simulink model "OpenSeesPy_Raspberry"  (R2021a)
settings: Solver=ode8  StartTime=0.0  StopTime=31.2  FixedStep=dtfast  RelTol=1e-3
PreLoadFcn:
  | initializeSimulation;
InitFcn:
  | clear('all');
  | initializeSimulation;
undefined symbols (not defined in the file): adaptive, Area, asiv, Be, Cl, denfilter, DiscIntNeverNeededParam, dtsim, fir_coef, forgfact, Gsnsr_DT, Gsnsr_FT, Kc, ke, kgap, khard, Kp, Kq, kv, learningrate, n1siv, n2siv, Ngap, nsiv, numfilter, P_corr_i, Seed_snr, ssAe, ssBe, ssCe, ssDe, stiffdeg, strdegHmos, tauv, V1, Vt, w_80, x02, xgap, xy
libraries: simulink x4, raspberrypiNetworklib x2
settings Model: Creator=diego.mera  LastModifiedBy=diego.mera
settings SolverCC: PositivePriorityOrder=on
settings OptimizationCC: EnhancedBackFolding=on  PassReuseOutputArgsAs=Individual arguments  ZeroExternalMemoryAtStartup=off  ZeroInternalMemoryAtStartup=off  MaxStackSize=64  OptimizeBlockOrder=speed  DifferentSizesBufferReuse=on  OptimizationCustomize=off  EfficientTunableParamExpr=on
settings DebuggingCC: ParameterTunabilityLossMsg=error
settings HardwareCC: ProdBitPerPointer=32  ProdBitPerSizeT=32  ProdBitPerPtrDiffT=32  ProdLargestAtomicInteger=Long  ProdLargestAtomicFloat=Double  ProdWordSize=32  ProdLongLongMode=on  ProdHWDeviceType=ARM Compatible->ARM Cortex
settings RTWCC: SystemTargetFile=ert.tlc  HardwareBoard=Raspberry Pi  TLCOptions="-aInlineSetEventsForThisBaseRateFcn=TLC_FALSE -aSuppressMultiTaskScheduler=TLC_FALSE  -aRateBasedStepFcn=0"  TemplateMakefile=ert_default_tmf  Toolchain=GNU GCC Embedded Linux  BuildConfiguration=Faster Runs
settings CodeAppCC: ForceParamTrailComments=on  IgnoreCustomStorageClasses=off  OperatorAnnotations=on  SimulinkDataObjDesc=on  SFDataObjDesc=on  InsertBlockDesc=on
settings ERTTargetCC: SupportContinuousTime=on  SupportVariableSizeSignals=on  ExtModeTransport=2  ExtModeStaticAlloc=on  ExtModeMexFile=ext_xcp  ExtModeIntrfLevel=Level2 - Open

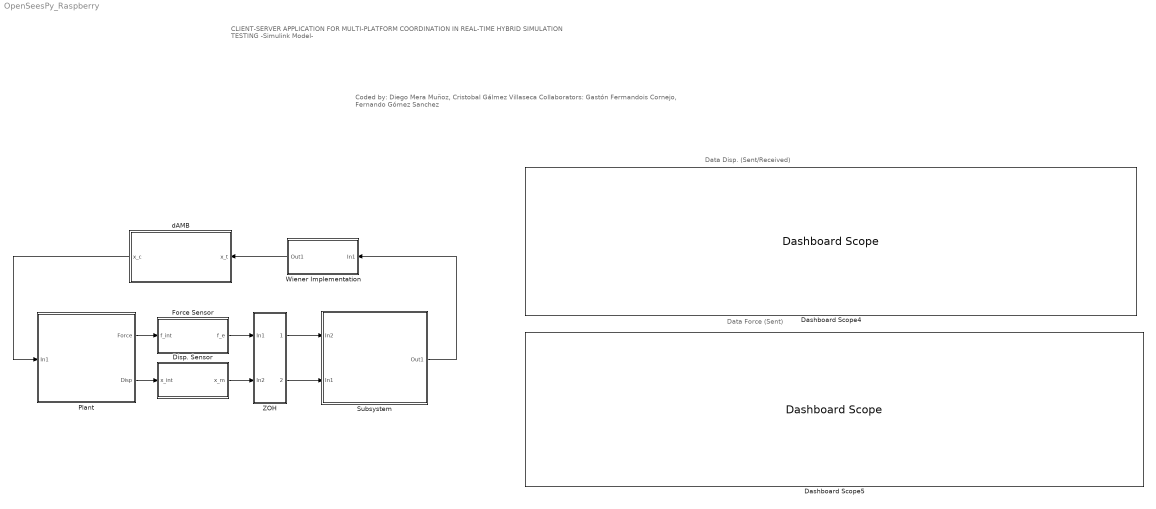
== system OpenSeesPy_Raspberry ==
  note: Data Disp. (Sent/Received)
  note: Data Force (Sent)
  note: Coded by: Diego Mera Muñoz, Cristobal Gálmez Villaseca
      | Collaborators: Gastón Fermandois Cornejo, Fernando Gómez Sanchez
  note: CLIENT-SERVER APPLICATION FOR MULTI-PLATFORM COORDINATION IN REAL-TIME HYBRID SIMULATION TESTING
      | -Simulink Model-
  Dashboard Scope4 : DashboardScope  Ymin=-5  Ymax=5
  Dashboard Scope5 : DashboardScope  Ymin=-1.5e-5  Ymax=1e-5
  Disp. Sensor : Subsystem
      mask Display: disp('DISP. SENSOR')
  Force Sensor : Subsystem
      mask Display: disp('FORCE SENSOR')
  Plant : Subsystem
      mask Display: disp('PLANT\n(Actuator-ES)')
  Subsystem : Subsystem
      mask Display: disp('NUMERICAL\nSUBSTRUCTURE')
  Wiener Implementation : Subsystem
      mask Display: disp('MBMRT FILTER')
  ZOH : Subsystem
      mask Display: disp('ZOH')
  dAMB : Subsystem
      mask Display: disp('DISCRETE ADAPTIVE\nMODEL-BASED\nCOMPENSATION')
  wires:
  Subsystem/1(Out1) -> Wiener Implementation/1(In1)
  Wiener Implementation/1(Out1) -> dAMB/1(x_t)
  Plant/1(Force) -> Force Sensor/1(f_int)
  Plant/2(Disp) -> Disp. Sensor/1(x_int)
  dAMB/1(x_c) -> Plant/1(In1)
  ZOH/1(Out1) -> Subsystem/1(In2)
  ZOH/2(Out2) -> Subsystem/2(In1)
  Force Sensor/1("f_e ") -> ZOH/1(In1)
  Disp. Sensor/1(x_m) -> ZOH/2(In2)

== system OpenSeesPy_Raspberry/Disp. Sensor ==
  x_int : Inport
  Sensor Noise : simulink/Sources/Band-Limited White Noise  Cov=rms_noise_DT  Ts=dtsim  seed=double(Seed_snr.Seed)
  Sensor Gain LVDT : Gain  Gain=Gsnsr_DT  SaturateOnIntegerOverflow=on  OutDataTypeStr=Inherit: Same as input  ParamDataTypeStr=Inherit: Same as input
  Sum : Sum  Inputs=|++  InputSameDT=on  SaturateOnIntegerOverflow=on  OutDataTypeStr=Inherit: Same as first input
  x_m : Outport
  tag scope: x_m=global
  wires:
  Sensor Noise/1 -> Sum/2
  Sum/1 -> x_m/1, [x_m]  "x_m"
  x_int/1 -> Sensor Gain LVDT/1
  Sensor Gain LVDT/1 -> Sum/1

== system OpenSeesPy_Raspberry/Force Sensor ==
  f_int : Inport
  Sensor Noise1 : simulink/Sources/Band-Limited White Noise  Cov=rms_noise_FT  Ts=dtsim  seed=double(Seed_snr.Seed)
  Sensor Gain LOAD CELL : Gain  Gain=Gsnsr_FT  SaturateOnIntegerOverflow=on  OutDataTypeStr=Inherit: Same as input  ParamDataTypeStr=Inherit: Same as input
  Sum1 : Sum  Inputs=|++  InputSameDT=on  SaturateOnIntegerOverflow=on  OutDataTypeStr=Inherit: Same as first input
  "f_e " : Outport
  wires:
  f_int/1 -> Sensor Gain LOAD CELL/1
  Sensor Noise1/1 -> Sum1/2
  Sum1/1 -> "f_e "/1
  Sensor Gain LOAD CELL/1 -> Sum1/1

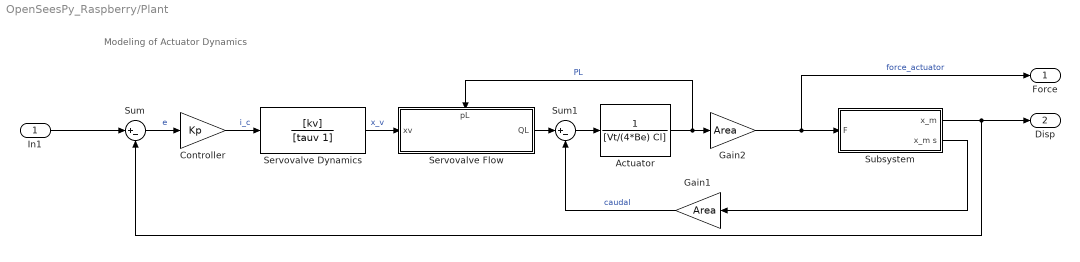
== system OpenSeesPy_Raspberry/Plant ==
  note: Modeling of Actuator Dynamics
  In1 : Inport
  Actuator : TransferFcn  Denominator=[Vt/(4*Be) Cl]
      mask Display: image(imread('actuator.PNG'));
  Controller : Gain  Gain=Kp
  Gain1 : Gain  Gain=Area
  Gain2 : Gain  Gain=Area
  Servovalve Dynamics : TransferFcn  Numerator=[kv]  Denominator=[tauv 1]
      mask Display: image(imread('servo2.PNG'));
  Servovalve Flow : Subsystem
      settings: PortSchema="{\"entries\":[{\"content\":{\"sides\":[{\"content\":{\"connectorIds\":[\"In1\"]},\"type\":\"ConnectorPlacement.EquallySpacedRectSide\",\"uuid\":\"f3a8b7d5-d784-462c-bc82-60644eee5a75\"},{\"content\":{\"connectorIds\":[\"Out1\"],\"side\":\"RIGHT\"},\"type\":\"ConnectorPlacement.EquallySpacedRectSide\",\"uuid\":\"5e6f1f83-a632-4bc9-a761-43cae998e77f\"},{\"content\":{\"connectorIds\":[\"In2\"],\"side\":\"TOP\"},\"type\":\"ConnectorPlacement.EquallySpacedRectSide\",\"uuid\":\"989b0903-e260-4847-946f-0ac5d5e511f7\"}]},\"type\":\"ConnectorPlacement.EquallySpacedConnector\",\"uuid\":\"5619e211-faa3-4076-b1a0-b20862ba0eaa\"}],\"packageUris\":[\"http://schema.mathworks.com/mf0/Connector/19700101\"],\"version\":\"1.0\"}"
      mask Display: image(imread('servo.PNG'));
  Subsystem : Subsystem
      mask Display: disp('EXPERIMENTAL\nSUBSTRUCTURE')
  Sum : Sum  Inputs=|+-
  Sum1 : Sum  Inputs=|+-
  Force : Outport
  Disp : Outport  Port=2
  wires:
  Sum/1 -> Controller/1  "e"
  Servovalve Dynamics/1 -> Servovalve Flow/1(xv)  "x_v"
  Gain1/1 -> Sum1/2  "caudal"
  Actuator/1 -> Servovalve Flow/2(pL), Gain2/1  "PL"
  Sum1/1 -> Actuator/1
  Controller/1 -> Servovalve Dynamics/1  "i_c"
  Servovalve Flow/1(QL) -> Sum1/1
  Gain2/1 -> Subsystem/1(F), Force/1  "force_actuator"
  Subsystem/2(x_m s) -> Gain1/1
  Subsystem/1(x_m) -> Disp/1, Sum/2
  In1/1 -> Sum/1

== system OpenSeesPy_Raspberry/Subsystem ==
  In2 : Inport
  In1 : Inport  Port=2
  Display10 : Display
  TCP/IP Receive2 : raspberrypiNetworklib/TCP//IP Receive  Priority=2  Mode_=Client  LocalServerPort_=8090  RemoteAddr_=192.168.0.18  RemoteServerPort_=8090  DataType_=double  DataSize_=1  SampleTime_=dtsim  SimulateUsing=Code generation  ClientPortBindingSelection_=off  ClientPortToBind_=35000  BlockingMode_=on  BlockTimeout_=0.01  BlockPlatform=RASPBERRYPI
      settings: SourceProductBaseCode=RASPPI
  TCP/IP Send1 : raspberrypiNetworklib/TCP//IP Send  Priority=1  Mode_=Client  LocalServerPort_=8090  RemoteAddr_=192.168.0.18  RemoteServerPort_=8090  SimulateUsing=Code generation  ClientPortBindingSelection_=off  ClientPortToBind_=35000  BlockingMode_=on  BlockTimeout_=0.02  BlockPlatform=RASPBERRYPI
      settings: SourceProductBaseCode=RASPPI
  Terminator : Terminator
  Out1 : Outport
  wires:
  In1/1 -> Terminator/1
  In2/1 -> TCP/IP Send1/1  "Disp_Num"
  TCP/IP Receive2/1 -> Out1/1
  TCP/IP Receive2/2 -> Display10/1

== system OpenSeesPy_Raspberry/Wiener Implementation ==
  In1 : Inport
  Prediction_Fixed_Adaptive : Subsystem
      mask Display: disp('PREDICTION\n(Adaptive/Fixed w)')
  Test3 : Subsystem
      mask Display: disp('MONOMIAL\nINTERPOLATION')
  To Workspace : ToWorkspace  VariableName=adaptive_parameters  SaveFormat=Timeseries  SampleTime=-1
  Out1 : Outport
  wires:
  Prediction_Fixed_Adaptive/2(Out2) -> To Workspace/1
  Test3/1(Out1) -> Out1/1
  In1/1 -> Prediction_Fixed_Adaptive/1(In1)
  Prediction_Fixed_Adaptive/1(Out1) -> Test3/1(In1)

== system OpenSeesPy_Raspberry/ZOH ==
  In1 : Inport
  In2 : Inport  Port=2
  Rate Transition : RateTransition  OutPortSampleTime=dtsim
  Rate Transition1 : RateTransition  OutPortSampleTime=dtsim
  Out1 : Outport
  Out2 : Outport  Port=2
  wires:
  In1/1 -> Rate Transition/1
  In2/1 -> Rate Transition1/1
  Rate Transition/1 -> Out1/1  "Force_Num"
  Rate Transition1/1 -> Out2/1  "Disp_Num"

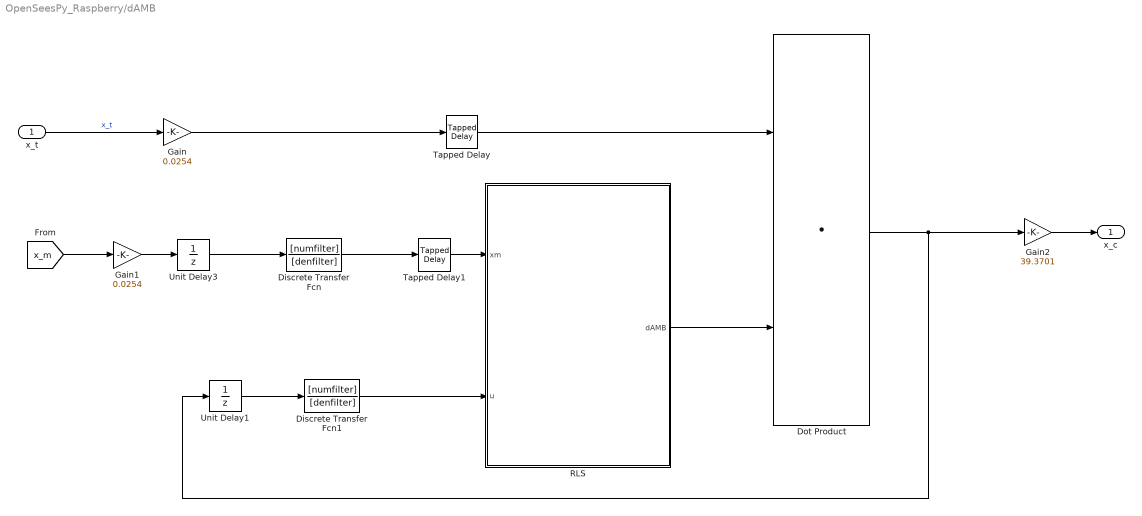
== system OpenSeesPy_Raspberry/dAMB ==
  x_t : Inport
  Discrete Transfer Fcn : DiscreteTransferFcn  Numerator=[numfilter]  Denominator=[denfilter]
  Discrete Transfer Fcn1 : DiscreteTransferFcn  Numerator=[numfilter]  Denominator=[denfilter]
  Dot Product : DotProduct  InputSameDT=on  OutDataTypeStr=Inherit: Inherit via internal rule
  Gain : Gain  Gain=0.0254
  Gain1 : Gain  Gain=0.0254
  Gain2 : Gain  Gain=39.3701
  RLS : Subsystem
  Tapped Delay : simulink/Discrete/Tapped Delay  vinit=0.0  samptime=-1  NumDelays=fir_coef-1  DelayOrder=Newest  includeCurrent=on
  Tapped Delay1 : simulink/Discrete/Tapped Delay  vinit=0.0  samptime=-1  NumDelays=fir_coef-1  DelayOrder=Newest  includeCurrent=on
  Unit Delay1 : UnitDelay  SampleTime=-1  HasFrameUpgradeWarning=on
  Unit Delay3 : UnitDelay  SampleTime=-1  HasFrameUpgradeWarning=on
  x_c : Outport  VectorParamsAs1DForOutWhenUnconnected=off
  wires:
  Gain1/1 -> Unit Delay3/1
  Gain/1 -> Tapped Delay/1
  Tapped Delay/1 -> Dot Product/1
  x_t/1 -> Gain/1  "x_t"
  Discrete Transfer Fcn/1 -> Tapped Delay1/1
  Discrete Transfer Fcn1/1 -> RLS/2(u)
  Tapped Delay1/1 -> RLS/1(xm)
  RLS/1(dAMB) -> Dot Product/2
  Unit Delay3/1 -> Discrete Transfer Fcn/1
  Unit Delay1/1 -> Discrete Transfer Fcn1/1
  Dot Product/1 -> Gain2/1, Unit Delay1/1
  Gain2/1 -> x_c/1
  [x_m] -> Gain1/1

== system OpenSeesPy_Raspberry/Plant/Servovalve Flow ==
  xv : Inport
  pL : Inport  Port=2
  Gain : Gain  Gain=Kq
  Gain1 : Gain  Gain=Kc
  Subtract : Sum  Inputs=+-
  QL : Outport
  wires:
  Gain1/1 -> Subtract/2
  pL/1 -> Gain1/1
  Subtract/1 -> QL/1
  Gain/1 -> Subtract/1
  xv/1 -> Gain/1

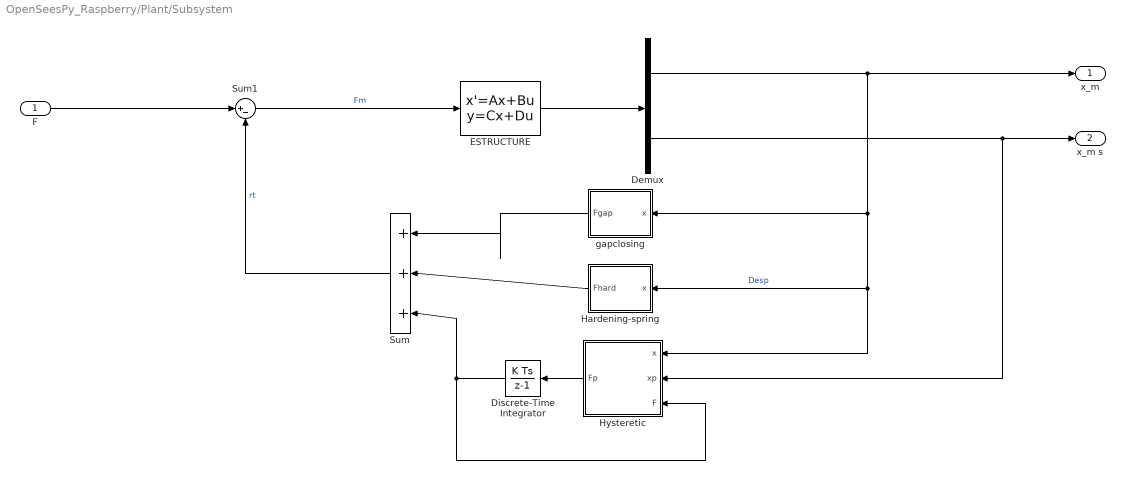
== system OpenSeesPy_Raspberry/Plant/Subsystem ==
  F : Inport
  Demux : Demux  Outputs=2
  Discrete-Time Integrator : DiscreteIntegrator  SampleTime=-1  ICPrevOutput=DiscIntNeverNeededParam  ICPrevScaledInput=DiscIntNeverNeededParam
  ESTRUCTURE : StateSpace  A=ssAe  B=ssBe  C=ssCe  D=ssDe  InitialCondition=0
  Hardening-spring : Subsystem
  Hysteretic : Subsystem
  Sum : Sum  Inputs=|+++
  Sum1 : Sum  Inputs=|+-
  gapclosing : Subsystem
  x_m : Outport  VectorParamsAs1DForOutWhenUnconnected=off
  x_m s : Outport  Port=2  VectorParamsAs1DForOutWhenUnconnected=off
  wires:
  Sum/1 -> Sum1/2  "rt"
  gapclosing/1(Fgap) -> Sum/1
  Sum1/1 -> ESTRUCTURE/1  "Fm"
  Discrete-Time Integrator/1 -> Sum/3, Hysteretic/3(F)
  Hardening-spring/1(Fhard) -> Sum/2
  Demux/1 -> x_m/1, Hardening-spring/1(x), Hysteretic/1(x), gapclosing/1(x)  "Desp"
  Hysteretic/1(Fp) -> Discrete-Time Integrator/1
  F/1 -> Sum1/1
  Demux/2 -> x_m s/1, Hysteretic/2(xp)
  ESTRUCTURE/1 -> Demux/1

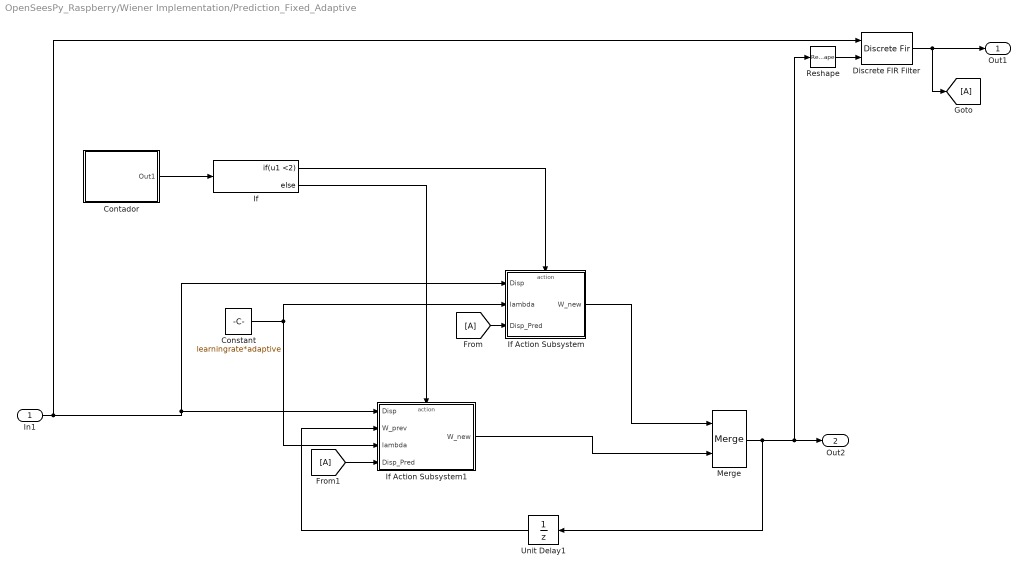
== system OpenSeesPy_Raspberry/Wiener Implementation/Prediction_Fixed_Adaptive ==
  In1 : Inport
  Constant : Constant  Value=learningrate*adaptive
  Contador : Subsystem
      mask Display: disp('Contador')
  Discrete FIR Filter : DiscreteFir  CoefSource=Input port  SampleTime=dtsim
      settings: InputPortMap=u0,u1
  If : If  IfExpression=u1 <2
  If Action Subsystem : Subsystem  TreatAsAtomicUnit=on
  If Action Subsystem1 : Subsystem  TreatAsAtomicUnit=on
  Merge : Merge
  Reshape : Reshape
  Unit Delay1 : UnitDelay  SampleTime=-1  HasFrameUpgradeWarning=on
  Out1 : Outport
  Out2 : Outport  Port=2
  wires:
  If Action Subsystem/1(W_new) -> Merge/1
  In1/1 -> Discrete FIR Filter/1, If Action Subsystem/1(Disp), If Action Subsystem1/1(Disp)
  If Action Subsystem1/1(W_new) -> Merge/2
  If/1 -> If Action Subsystem/Action
  Unit Delay1/1 -> If Action Subsystem1/2(W_prev)
  Merge/1 -> Reshape/1, Out2/1, Unit Delay1/1
  If/2 -> If Action Subsystem1/Action
  Contador/1(Out1) -> If/1
  Constant/1 -> If Action Subsystem1/3(lambda), If Action Subsystem/2(lambda)
  Discrete FIR Filter/1 -> [A], Out1/1
  [A] -> If Action Subsystem/3(Disp_Pred)
  [A] -> If Action Subsystem1/4(Disp_Pred)
  Reshape/1 -> Discrete FIR Filter/2

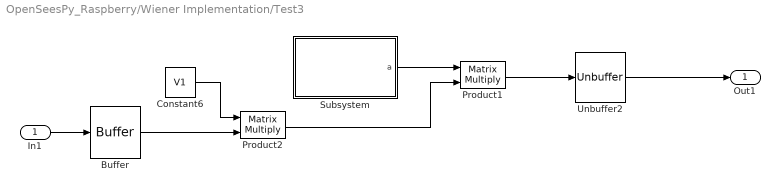
== system OpenSeesPy_Raspberry/Wiener Implementation/Test3 ==
  In1 : Inport
  Buffer : Buffer  N=4  V=3  OutputFrames=off
  Constant6 : Constant  Value=V1
  Product1 : Product  Multiplication=Matrix(*)
  Product2 : Product  Multiplication=Matrix(*)
  Subsystem : Subsystem
  Unbuffer2 : Unbuffer
  Out1 : Outport
  wires:
  Product2/1 -> Product1/2
  Constant6/1 -> Product2/1
  Unbuffer2/1 -> Out1/1
  In1/1 -> Buffer/1
  Product1/1 -> Unbuffer2/1
  Subsystem/1(a) -> Product1/1
  Buffer/1 -> Product2/2

== system OpenSeesPy_Raspberry/dAMB/RLS ==
  xm : Inport
  u : Inport  Port=2
  Constant6 : Constant  Value=forgfact
  Delay1 : Delay  DelayLength=1  InitialCondition=P_corr_i
  Delay2 : Delay  DelayLength=1  InitialCondition=dAMB_i'
  RLS : MATLAB Function  TreatAsAtomicUnit=on
  dAMB : Outport  VectorParamsAs1DForOutWhenUnconnected=off
  wires:
  xm/1 -> RLS/1(xm)
  Delay2/1 -> RLS/4(dAMB_a)
  u/1 -> RLS/2(u)
  RLS/2(P_corr) -> Delay1/1  "P_corr"
  Delay1/1 -> RLS/5(P_corr_a)
  Constant6/1 -> RLS/3(forgfact)
  RLS/1(dAMB) -> Delay2/1, dAMB/1  "dAMB"

== system OpenSeesPy_Raspberry/Plant/Subsystem/Hardening-spring ==
  x : Inport
  Constant1 : Constant  Value=khard
  MATLAB Function : MATLAB Function  TreatAsAtomicUnit=on
  Unit Delay : UnitDelay  SampleTime=-1  HasFrameUpgradeWarning=on
  Fhard : Outport  VectorParamsAs1DForOutWhenUnconnected=off
  wires:
  x/1 -> Unit Delay/1
  Constant1/1 -> MATLAB Function/2(khard)
  MATLAB Function/1(Fhard) -> Fhard/1
  Unit Delay/1 -> MATLAB Function/1(x)

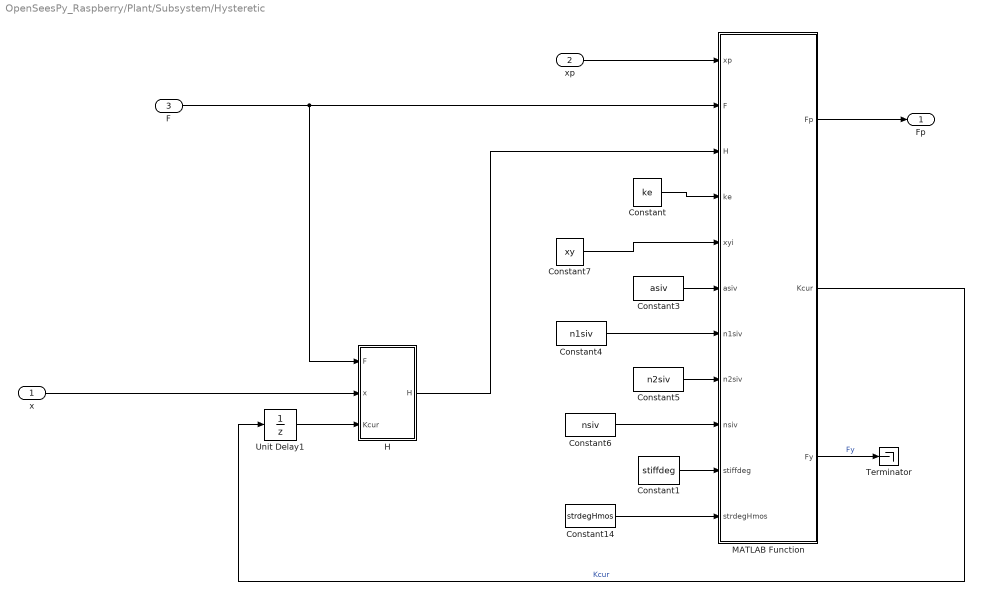
== system OpenSeesPy_Raspberry/Plant/Subsystem/Hysteretic ==
  x : Inport
  xp : Inport  Port=2
  F : Inport  Port=3
  Constant : Constant  Value=ke
  Constant1 : Constant  Value=stiffdeg
  Constant14 : Constant  Value=strdegHmos
  Constant3 : Constant  Value=asiv
  Constant4 : Constant  Value=n1siv
  Constant5 : Constant  Value=n2siv
  Constant6 : Constant  Value=nsiv
  Constant7 : Constant  Value=xy
  H : Subsystem
  MATLAB Function : MATLAB Function  TreatAsAtomicUnit=on
  Terminator : Terminator
  Unit Delay1 : UnitDelay  InitialCondition=ke  SampleTime=-1  HasFrameUpgradeWarning=on
  Fp : Outport  VectorParamsAs1DForOutWhenUnconnected=off
  wires:
  MATLAB Function/1(Fp) -> Fp/1
  MATLAB Function/2(Kcur) -> Unit Delay1/1  "Kcur"
  x/1 -> H/2(x)
  xp/1 -> MATLAB Function/1(xp)
  Constant/1 -> MATLAB Function/4(ke)
  Constant7/1 -> MATLAB Function/5(xyi)
  Constant1/1 -> MATLAB Function/10(stiffdeg)
  Constant3/1 -> MATLAB Function/6(asiv)
  Constant4/1 -> MATLAB Function/7(n1siv)
  Constant5/1 -> MATLAB Function/8(n2siv)
  Constant6/1 -> MATLAB Function/9(nsiv)
  H/1(H) -> MATLAB Function/3(H)
  Unit Delay1/1 -> H/3("Kcur ")
  F/1 -> MATLAB Function/2(F), H/1(F)
  Constant14/1 -> MATLAB Function/11(strdegHmos)
  MATLAB Function/3(Fy) -> Terminator/1  "Fy"

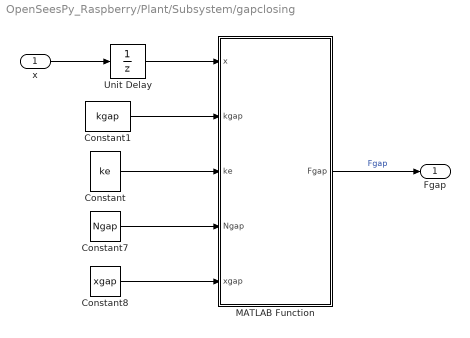
== system OpenSeesPy_Raspberry/Plant/Subsystem/gapclosing ==
  x : Inport
  Constant : Constant  Value=ke
  Constant1 : Constant  Value=kgap
  Constant7 : Constant  Value=Ngap
  Constant8 : Constant  Value=xgap
  MATLAB Function : MATLAB Function  TreatAsAtomicUnit=on
  Unit Delay : UnitDelay  SampleTime=-1  HasFrameUpgradeWarning=on
  Fgap : Outport  VectorParamsAs1DForOutWhenUnconnected=off
  wires:
  Constant7/1 -> MATLAB Function/4(Ngap)
  MATLAB Function/1(Fgap) -> Fgap/1  "Fgap"
  Constant1/1 -> MATLAB Function/2(kgap)
  Constant8/1 -> MATLAB Function/5(xgap)
  Constant/1 -> MATLAB Function/3(ke)
  x/1 -> Unit Delay/1
  Unit Delay/1 -> MATLAB Function/1(x)

== system OpenSeesPy_Raspberry/Wiener Implementation/Prediction_Fixed_Adaptive/Contador ==
  Add : Sum
  Constant1 : Constant
  Unit Delay : UnitDelay  SampleTime=-1  HasFrameUpgradeWarning=on
  Out1 : Outport
  wires:
  Unit Delay/1 -> Add/2
  Constant1/1 -> Add/1
  Add/1 -> Out1/1, Unit Delay/1

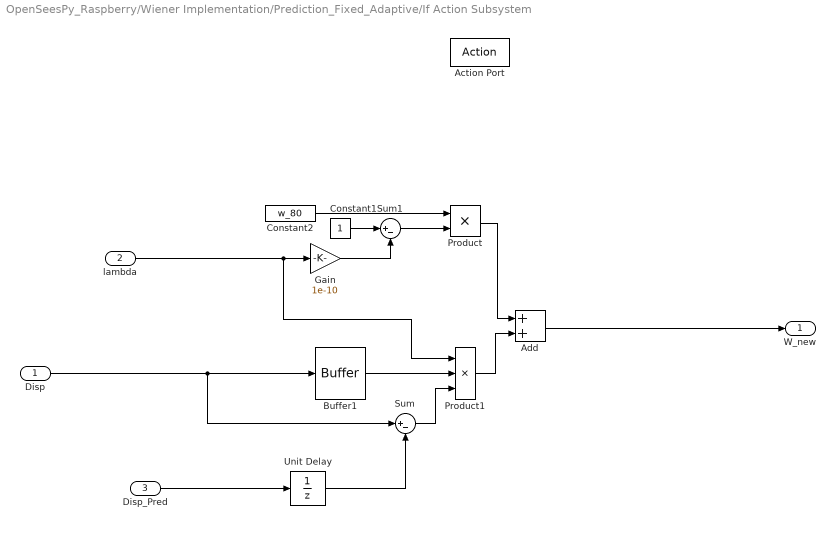
== system OpenSeesPy_Raspberry/Wiener Implementation/Prediction_Fixed_Adaptive/If Action Subsystem ==
  Disp : Inport
  lambda : Inport  Port=2
  Disp_Pred : Inport  Port=3
  Action Port : ActionPort  ActionPortLabel=if(u1 <2)
  Add : Sum
  Buffer1 : Buffer  N=8  V=7  OutputFrames=off
  Constant1 : Constant
  Constant2 : Constant  Value=w_80
  Gain : Gain  Gain=1e-10
  Product : Product
  Product1 : Product  Inputs=3
  Sum : Sum  Inputs=|+-
  Sum1 : Sum  Inputs=|+-
  Unit Delay : UnitDelay  SampleTime=-1  HasFrameUpgradeWarning=on
  W_new : Outport
  wires:
  lambda/1 -> Product1/1, Gain/1
  Gain/1 -> Sum1/2
  Add/1 -> W_new/1
  Constant2/1 -> Product/1
  Buffer1/1 -> Product1/2
  Product1/1 -> Add/2
  Product/1 -> Add/1
  Disp/1 -> Buffer1/1, Sum/1
  Sum1/1 -> Product/2
  Sum/1 -> Product1/3
  Unit Delay/1 -> Sum/2
  Constant1/1 -> Sum1/1
  Disp_Pred/1 -> Unit Delay/1

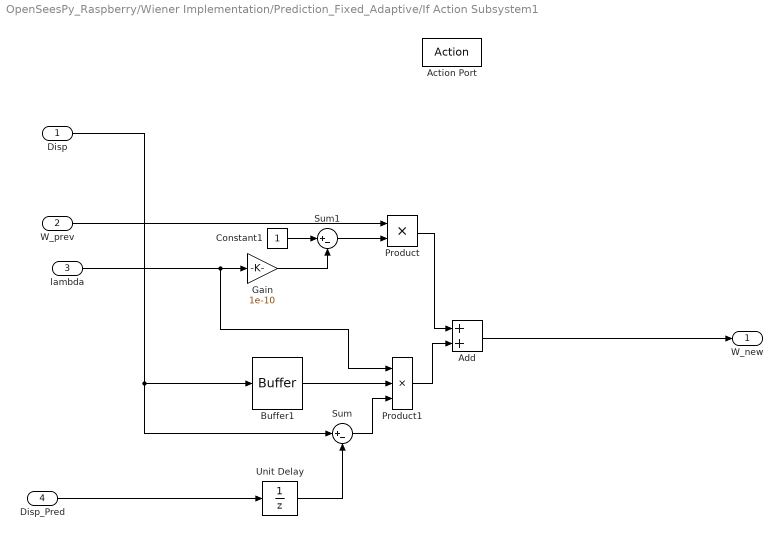
== system OpenSeesPy_Raspberry/Wiener Implementation/Prediction_Fixed_Adaptive/If Action Subsystem1 ==
  Disp : Inport
  W_prev : Inport  Port=2
  lambda : Inport  Port=3
  Disp_Pred : Inport  Port=4
  Action Port : ActionPort  ActionPortLabel=else
  Add : Sum
  Buffer1 : Buffer  N=8  V=7  OutputFrames=off
  Constant1 : Constant
  Gain : Gain  Gain=1e-10
  Product : Product
  Product1 : Product  Inputs=3
  Sum : Sum  Inputs=|+-
  Sum1 : Sum  Inputs=|+-
  Unit Delay : UnitDelay  SampleTime=-1  HasFrameUpgradeWarning=on
  W_new : Outport
  wires:
  lambda/1 -> Product1/1, Gain/1
  Gain/1 -> Sum1/2
  Add/1 -> W_new/1
  W_prev/1 -> Product/1
  Buffer1/1 -> Product1/2
  Product1/1 -> Add/2
  Product/1 -> Add/1
  Disp/1 -> Buffer1/1, Sum/1
  Sum1/1 -> Product/2
  Sum/1 -> Product1/3
  Unit Delay/1 -> Sum/2
  Constant1/1 -> Sum1/1
  Disp_Pred/1 -> Unit Delay/1

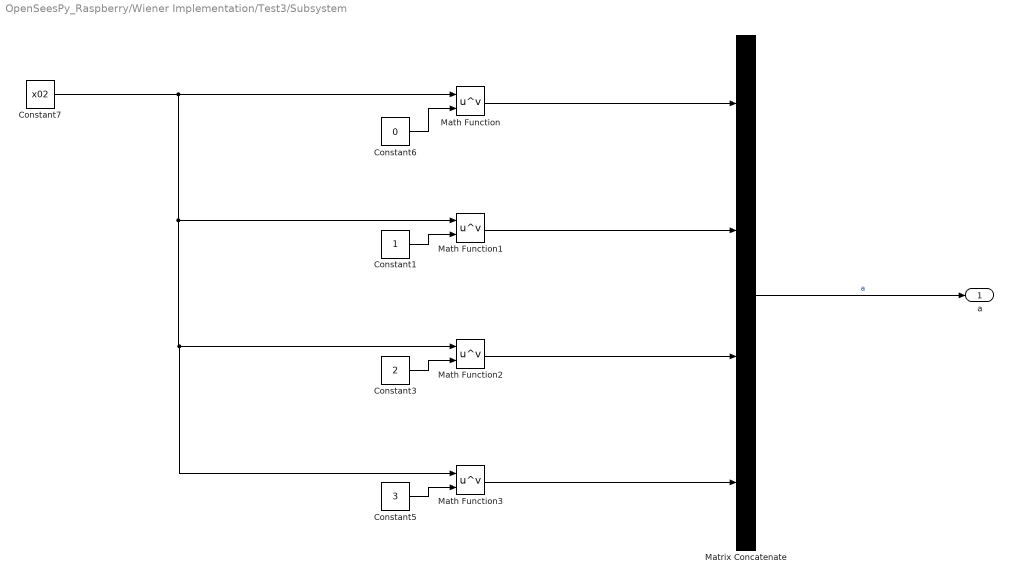
== system OpenSeesPy_Raspberry/Wiener Implementation/Test3/Subsystem ==
  Constant1 : Constant
  Constant3 : Constant  Value=2
  Constant5 : Constant  Value=3
  Constant6 : Constant  Value=0
  Constant7 : Constant  Value=x02
  Math Function{,1..3} (4 alike) : Math  Operator=pow  SaturateOnIntegerOverflow=on
  Matrix Concatenate : Concatenate  NumInputs=4  Mode=Multidimensional array  ConcatenateDimension=2
  a : Outport
  wires:
  Constant6/1 -> Math Function/2
  Constant1/1 -> Math Function1/2
  Constant3/1 -> Math Function2/2
  Constant5/1 -> Math Function3/2
  Math Function/1 -> Matrix Concatenate/1
  Math Function1/1 -> Matrix Concatenate/2
  Math Function2/1 -> Matrix Concatenate/3
  Math Function3/1 -> Matrix Concatenate/4
  Matrix Concatenate/1 -> a/1  "a"
  Constant7/1 -> Math Function3/1, Math Function2/1, Math Function1/1, Math Function/1

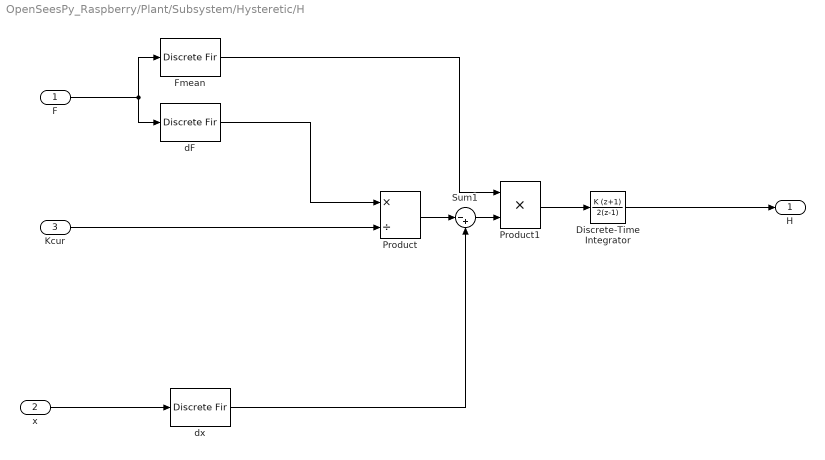
== system OpenSeesPy_Raspberry/Plant/Subsystem/Hysteretic/H ==
  F : Inport
  x : Inport  Port=2
  "Kcur " : Inport  Port=3
  Discrete-Time Integrator : DiscreteIntegrator  IntegratorMethod=Accumulation: Trapezoidal  SampleTime=-1  ICPrevOutput=DiscIntNeverNeededParam  ICPrevScaledInput=DiscIntNeverNeededParam
  Fmean : DiscreteFir
  Product : Product  Inputs=*/
  Product1 : Product
  Sum1 : Sum  Inputs=|-+
  dF : DiscreteFir  Coefficients=[1 -1]
  dx : DiscreteFir  Coefficients=[1 -1]
  H : Outport  VectorParamsAs1DForOutWhenUnconnected=off
  wires:
  dF/1 -> Product/1
  "Kcur "/1 -> Product/2
  Product1/1 -> Discrete-Time Integrator/1
  Sum1/1 -> Product1/2
  x/1 -> dx/1
  F/1 -> Fmean/1, dF/1
  Discrete-Time Integrator/1 -> H/1
  Product/1 -> Sum1/1
  dx/1 -> Sum1/2
  Fmean/1 -> Product1/1

== matlab function OpenSeesPy_Raspberry/dAMB/RLS/RLS ==
  data: xm input; u input; forgfact input; dAMB_a input; P_corr_a input; dAMB output; P_corr output
function [dAMB,P_corr]  = fcn(xm,u,forgfact,dAMB_a,P_corr_a)             
        error=(u-dAMB_a'*xm);
        phik=P_corr_a*xm/(forgfact+xm'*P_corr_a*xm);
        P_corr=(P_corr_a-phik*xm'*P_corr_a)/forgfact;
        
        dAMB=dAMB_a+phik*error;
end

== matlab function OpenSeesPy_Raspberry/Plant/Subsystem/Hardening-spring/MATLAB Function ==
  data: x input; Fhard output; khard input
function Fhard  = hardening(x,khard)
Fhard=khard*(x^3);

== matlab function OpenSeesPy_Raspberry/Plant/Subsystem/Hysteretic/MATLAB Function ==
  data: xp input; F input; H input; Fp output; ke input; xyi input; asiv input; n1siv input; n2siv input; nsiv input; stiffdeg input; Kcur output; Fy output; strdegHmos input
function [Fp,Kcur,Fy] = stiffdegradation(xp,F,H,ke,xyi,asiv,n1siv,n2siv,nsiv,stiffdeg,strdegHmos)

Kcur=((exp(-stiffdeg*H))-asiv)*ke; 
Fyi=(1-asiv)*ke*xyi;
Fy=Fyi*(1+strdegHmos*H)^-1;
if Fy<=0.01*Fyi
    Fy=Fyi*0.01;
end
Khyst=Kcur*(1-abs(F/Fy)^(nsiv)*(n1siv*sign(F*xp)+n2siv));
Fp=Khyst*xp;

== matlab function OpenSeesPy_Raspberry/Plant/Subsystem/gapclosing/MATLAB Function ==
  data: x input; Fgap output; kgap input; ke input; Ngap input; xgap input
function Fgap  = gapclosing(x,kgap,ke,Ngap,xgap)
if abs(x)<=xgap
    Fgap=0;
else
    Fgap=kgap*ke*Ngap*(abs(x)-xgap)^(Ngap-1)*x;
end
